simulink model "class16"  (R2025b)
settings: Solver=VariableStepAuto  StartTime=0.0  StopTime=10.0  RelTol=1e-3
settings Model: Creator=anish  LastModifiedBy=anish

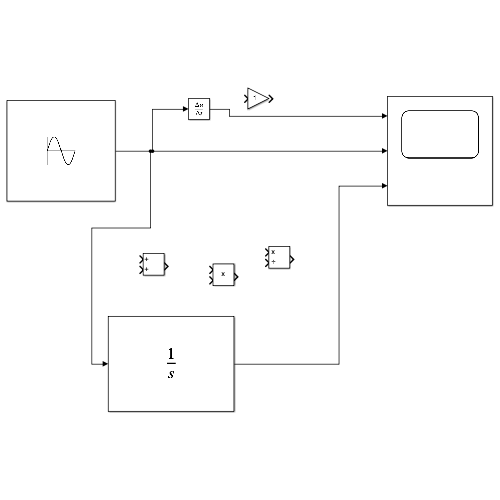
[thumbnail: Simulink's stored preview of the top-level diagram]
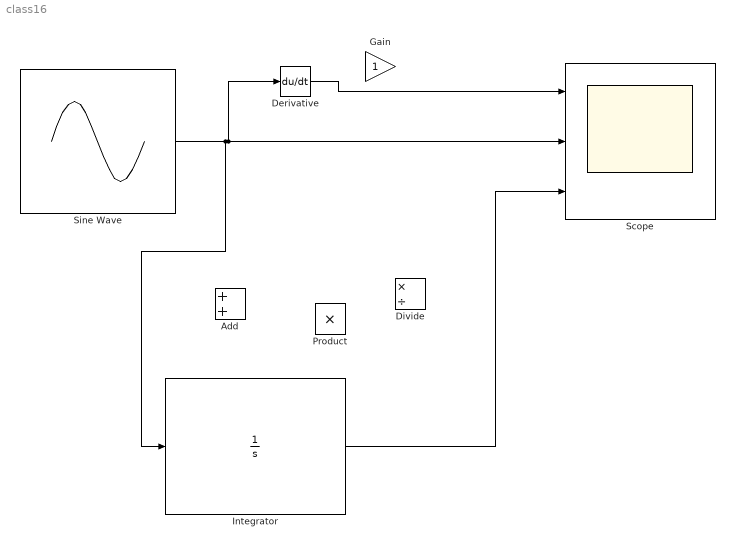
== system class16 ==
  Add : Sum
  Derivative : Derivative
  Divide : Product  Inputs=*/
  Gain : Gain
  Integrator : Integrator
  Product : Product
  Scope : Scope  NumInputPorts=3
      settings: SampleTime=0.01  ActiveDisplayYMinimum=-2.4075110831514679  ActiveDisplayYMaximum=3.6158186168691233
  Sine Wave : Sin  SampleTime=0
  wires:
  Derivative/1 -> Scope/1
  Sine Wave/1 -> Scope/2, Derivative/1, Integrator/1
  Integrator/1 -> Scope/3
